simulink model "hostModel"  (R2023b)
settings: Solver=FixedStepDiscrete  StartTime=0.0  StopTime=inf  RelTol=1e-3  EnableMultiTasking=on
InitFcn:
  | mcb_bldc_sixstep_f28069mLaunchPad_data;
StopFcn:
  | dataMonitoringArr;
values from neighbouring files (symbols this model uses):
  inverter = mcb_SetInverterParameters('SBLMB500')    [mcb_bldc_sixstep_f28069mLaunchPad_data.m]
  PU_System = mcb_SetPUSystem(bldc,inverter)    [mcb_bldc_sixstep_f28069mLaunchPad_data.m]
  Ts = 0.03    [dataMonitoringArr.m]    (also in mcb_bldc_sixstep_f28069mLaunchPad_data.m = 5e-05)
libraries: dspstat3 x5, instrumentseriallib x4
settings Model: Creator=The MathWorks, Inc.  LastModifiedBy=Tefilus
settings SolverCC: AlgebraicLoopSolver=TrustRegion  AutoInsertRateTranBlk=on  MaxZcPerStep=1
settings DataIOCC: LimitDataPoints=on  ReturnWorkspaceOutputs=off
settings OptimizationCC: ReuseModelBlockBuffer=off  LifeSpan=1  EfficientTunableParamExpr=on
settings DebuggingCC: UnderspecifiedInitializationDetection=Classic  MergeDetectMultiDrivingBlocksExec=none  SolverPrmCheckMsg=warning  ParameterPrecisionLossMsg=none  UnconnectedInputMsg=warning  UnconnectedOutputMsg=warning  UnconnectedLineMsg=warning  AllowSymbolicDim=off  PregeneratedLibrarySubsystemCodeDiagnostic=none  SFUnexpectedBacktrackingDiag=warning  SFNoUnconditionalDefaultTransitionDiag=warning  SFExecutionAtInitializationDiag=none  ArithmeticOperatorsInVariantConditions=warning
settings HardwareCC: ProdBitPerPointer=32  ProdLargestAtomicFloat=None  ProdIntDivRoundTo=Undefined  ProdEndianess=Unspecified  ProdWordSize=32  ProdHWDeviceType=32-bit Generic
settings ModelReferenceCC: EnableRefExpFcnMdlSchedulingChecks=on  PropagateSignalLabelsOutOfModel=off
settings SFSimCC: SimUseLocalCustomCode=off
settings RTWCC: Description=Real-Time Workshop Embedded Coder  SystemTargetFile=ert.tlc  TemplateMakefile=ert_default_tmf  GenerateReport=on  RTWUseLocalCustomCode=off  IncludeHyperlinkInReport=on  LaunchReport=on  GenerateTraceInfo=on  GenerateTraceReport=on  GenerateTraceReportSl=on  GenerateTraceReportSf=on  GenerateTraceReportEml=on  DLArmComputeVersion=19.05
settings CodeAppCC: IgnoreCustomStorageClasses=off  StateflowObjectComments=on  InternalIdentifier=Classic
settings ERTTargetCC: MultiwordLength=2048  GenerateSampleERTMain=on  ERTCustomFileTemplate=example_file_process.tlc  ConvertIfToSwitch=off  SuppressUnreachableDefaultCases=off
settings ConfigComp: CovMetricSettings=dw  CovSaveCumulativeToWorkspaceVar=on  CovSaveSingleToWorkspaceVar=on  CovExternalEMLEnable=off  CovSFcnEnable=off

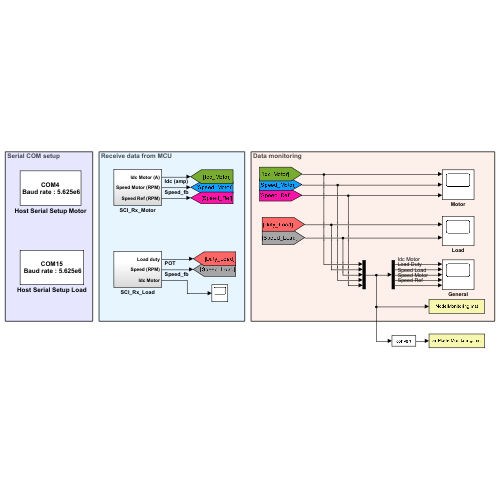
[thumbnail: Simulink's stored preview of the top-level diagram]
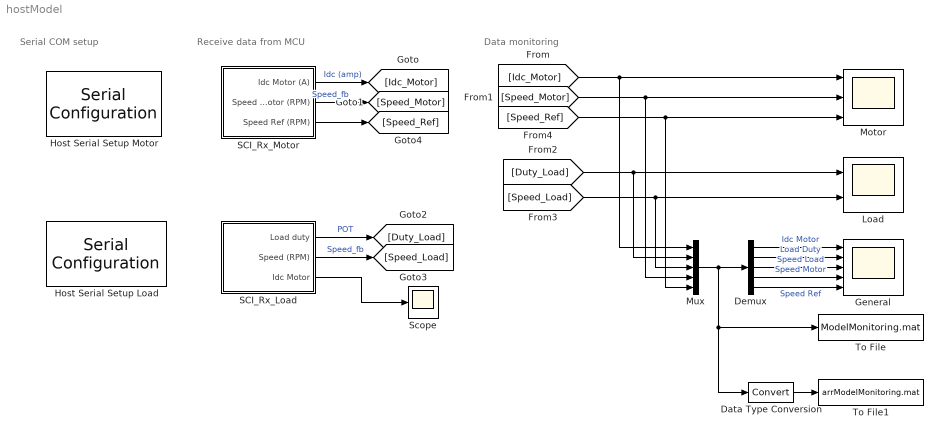
== system hostModel ==
  note: Serial COM setup
  note: Receive data from MCU
  note: Data monitoring
  Data Type Conversion : DataTypeConversion  SaturateOnIntegerOverflow=off  RndMeth=Floor
  Demux : Demux  Outputs=5
  General : Scope  NumInputPorts=5
  Host Serial Setup Load : instrumentseriallib/Serial Configuration  Priority=-99  PortSel=COM15  Port=COM15  ComPort=COM15  BaudRate=5.625e6  DataBits=8  Parity=none  StopBits=1  ByteOrder=little-endian  FlowControl=none  Timeout=2  SimulateUsing=Interpreted execution  BlockInModel=on  aMode=5
  Host Serial Setup Motor : instrumentseriallib/Serial Configuration  Priority=-99  PortSel=target.comport  Port=target.comport  ComPort=target.comport  BaudRate=5.625e6  DataBits=8  Parity=none  StopBits=1  ByteOrder=little-endian  FlowControl=none  Timeout=2  SimulateUsing=Interpreted execution  BlockInModel=on  aMode=5
  Load : Scope  NumInputPorts=2
  Motor : Scope  NumInputPorts=3
  Mux : Mux  Inputs=5
  SCI_Rx_Load : Subsystem
  SCI_Rx_Motor : Subsystem
  Scope : Scope
  To File : ToFile  Filename=ModelMonitoring.mat  MatrixName=IdcMtr_PotLd_SpMtr_SpLd  SaveFormat=Timeseries
  To File1 : ToFile  Filename=arrModelMonitoring.mat  MatrixName=IdcMtr_PotLd_SpMtr_SpLd
  wires:
  SCI_Rx_Motor/1(Idc Motor (A)) -> [Idc_Motor]  "Idc (amp)"
  SCI_Rx_Motor/2(Speed Motor (RPM)) -> [Speed_Motor]  "Speed_fb"
  SCI_Rx_Load/1(Load duty) -> [Duty_Load]  "POT"
  SCI_Rx_Load/2(Speed (RPM)) -> [Speed_Load]  "Speed_fb"
  [Idc_Motor] -> Mux/1, Motor/1
  [Duty_Load] -> Load/1, Mux/2
  [Speed_Load] -> Mux/3, Load/2
  Mux/1 -> To File/1, Data Type Conversion/1, Demux/1
  Demux/3 -> General/3  "Speed Load"
  Demux/4 -> General/4  "Speed Motor"
  Demux/2 -> General/2  "Load Duty"
  Demux/1 -> General/1  "Idc Motor"
  SCI_Rx_Motor/3(Speed Ref (RPM)) -> [Speed_Ref]
  [Speed_Motor] -> Mux/4, Motor/2
  [Speed_Ref] -> Mux/5, Motor/3
  Demux/5 -> General/5  "Speed Ref"
  SCI_Rx_Load/3(Idc Motor) -> Scope/1
  Data Type Conversion/1 -> To File1/1

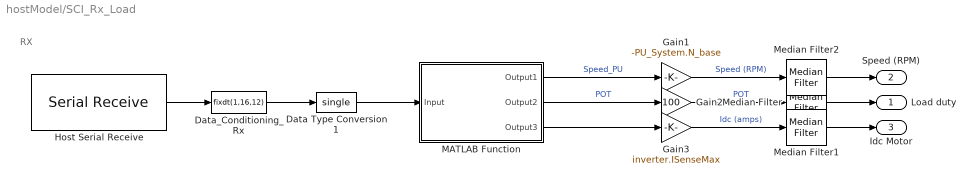
== system hostModel/SCI_Rx_Load ==
  note: RX
  Data Type Conversion1 : DataTypeConversion  OutDataTypeStr=single  RndMeth=Simplest  SaturateOnIntegerOverflow=off
  Data_Conditioning_Rx : DataTypeConversion  OutDataTypeStr=fixdt(1,16,12)  ConvertRealWorld=Stored Integer (SI)  RndMeth=Simplest  SaturateOnIntegerOverflow=off
  Gain1 : Gain  Gain=-PU_System.N_base  OutDataTypeStr=single  RndMeth=Simplest
  Gain2 : Gain  Gain=100  OutDataTypeStr=single  RndMeth=Simplest
  Gain3 : Gain  Gain=inverter.ISenseMax  OutDataTypeStr=single  RndMeth=Simplest
  Host Serial Receive : instrumentseriallib/Serial Receive  PortSel=COM15  Port=COM15  ComPort=COM15  DataType=uint16  SaveDataType=uint8  ToggleHeader=on  Header='SS'  ToggleTerminator=on  Terminator=Custom terminator  CustomTerminator='EE'  InputFormat=Row major  ToggleDataSize=on  DataSize=[600 3]  EnableBlockingMode=on  ActionDataUnavailable=Output last received value  ActionWhenDataUnavailable=Output last received value  CustomValue=0  SampleTime=600 * Ts  SimulateUsing=Interpreted execution  BlockInModel=on  aMode=5
  MATLAB Function : MATLAB Function  TreatAsAtomicUnit=on
  Median Filter : dspstat3/Median Filter  WindowLength=1001  SimulateUsing=Interpreted execution
      settings: LibrarySourceBlock=|
      | dspfdesign/Median
      | Filter
  Median Filter1 : dspstat3/Median Filter  WindowLength=5  SimulateUsing=Interpreted execution
      settings: LibrarySourceBlock=|
      | dspfdesign/Median
      | Filter
  Median Filter2 : dspstat3/Median Filter  WindowLength=5  SimulateUsing=Interpreted execution
      settings: LibrarySourceBlock=|
      | dspfdesign/Median
      | Filter
  Load duty : Outport
  Speed (RPM) : Outport  Port=2
  Idc Motor : Outport  Port=3
  wires:
  Host Serial Receive/1 -> Data_Conditioning_Rx/1
  MATLAB Function/1(Output1) -> Gain1/1  "Speed_PU"
  Data_Conditioning_Rx/1 -> Data Type Conversion1/1
  Data Type Conversion1/1 -> MATLAB Function/1(Input)
  Median Filter/1 -> Load duty/1
  Gain2/1 -> Median Filter/1  "POT"
  MATLAB Function/2(Output2) -> Gain2/1  "POT"
  MATLAB Function/3(Output3) -> Gain3/1
  Gain3/1 -> Median Filter1/1  "Idc (amps)"
  Median Filter1/1 -> Idc Motor/1
  Gain1/1 -> Median Filter2/1  "Speed (RPM)"
  Median Filter2/1 -> Speed (RPM)/1

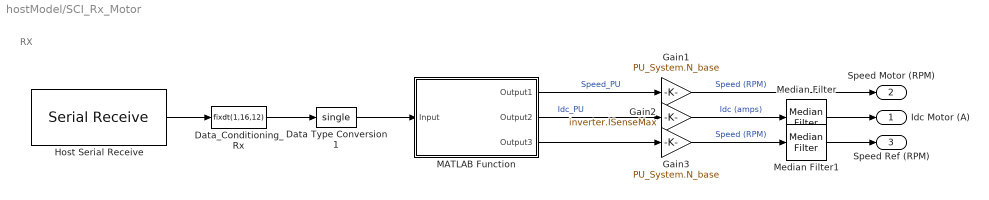
== system hostModel/SCI_Rx_Motor ==
  note: RX
  Data Type Conversion1 : DataTypeConversion  OutDataTypeStr=single  RndMeth=Simplest  SaturateOnIntegerOverflow=off
  Data_Conditioning_Rx : DataTypeConversion  OutDataTypeStr=fixdt(1,16,12)  ConvertRealWorld=Stored Integer (SI)  RndMeth=Simplest  SaturateOnIntegerOverflow=off
  Gain1 : Gain  Gain=PU_System.N_base  OutDataTypeStr=single  RndMeth=Simplest
  Gain2 : Gain  Gain=inverter.ISenseMax  OutDataTypeStr=single  RndMeth=Simplest
  Gain3 : Gain  Gain=PU_System.N_base  OutDataTypeStr=single  RndMeth=Simplest
  Host Serial Receive : instrumentseriallib/Serial Receive  PortSel=target.comport  Port=target.comport  ComPort=target.comport  DataType=uint16  SaveDataType=uint8  ToggleHeader=on  Header='SS'  ToggleTerminator=on  Terminator=Custom terminator  CustomTerminator='EE'  InputFormat=Row major  ToggleDataSize=on  DataSize=[600 3]  EnableBlockingMode=on  ActionDataUnavailable=Output last received value  ActionWhenDataUnavailable=Output last received value  CustomValue=0  SampleTime=600 * Ts  SimulateUsing=Interpreted execution  BlockInModel=on  aMode=5
  MATLAB Function : MATLAB Function  TreatAsAtomicUnit=on
  Median Filter : dspstat3/Median Filter  WindowLength=1001  SimulateUsing=Interpreted execution
      settings: LibrarySourceBlock=|
      | dspfdesign/Median
      | Filter
  Median Filter1 : dspstat3/Median Filter  WindowLength=101  SimulateUsing=Interpreted execution
      settings: LibrarySourceBlock=|
      | dspfdesign/Median
      | Filter
  Idc Motor (A) : Outport
  Speed Motor (RPM) : Outport  Port=2
  Speed Ref (RPM) : Outport  Port=3
  wires:
  Host Serial Receive/1 -> Data_Conditioning_Rx/1
  MATLAB Function/1(Output1) -> Gain1/1  "Speed_PU"
  Data_Conditioning_Rx/1 -> Data Type Conversion1/1
  Data Type Conversion1/1 -> MATLAB Function/1(Input)
  Median Filter/1 -> Idc Motor (A)/1
  Gain2/1 -> Median Filter/1  "Idc (amps)"
  MATLAB Function/2(Output2) -> Gain2/1  "Idc_PU"
  MATLAB Function/3(Output3) -> Gain3/1
  Gain3/1 -> Median Filter1/1  "Speed (RPM)"
  Median Filter1/1 -> Speed Ref (RPM)/1
  Gain1/1 -> Speed Motor (RPM)/1  "Speed (RPM)"

== matlab function hostModel/SCI_Rx_Load/MATLAB Function ==
  data: Output1 output; Output2 output; Input input; Output3 output
function [ Output1, Output2, Output3] = unBuf(Input)

Output1 = Input(:, 1);
Output2 = Input(:, 2);
Output3 = Input(:, 3);
% Output4 = Input(:, 4);
end

== matlab function hostModel/SCI_Rx_Motor/MATLAB Function ==
  data: Output1 output; Output2 output; Input input; Output3 output
function [ Output1, Output2, Output3] = unBuf(Input)

Output1 = Input(:, 1);
Output2 = Input(:, 2);
Output3 = Input(:, 3);
% Output4 = Input(:, 4);
end
